simulink library "csu_itu_inertial_time_update_lib"  (R2014b)
settings: Solver=ode45  SolverMode=SingleTasking  StartTime=0.0  StopTime=10.0  RelTol=1e-3
values from neighbouring files (symbols this model uses):
  tup_process_noise_high = diag([1.1 1.1 10.1 , 0.000505   0.000505   0.000505 ,  0.00001 0.00001 0.00001 , 0.001 0.001 0.001 , 0.001 0.001 0.001 ])    [csc_tup_time_update_init.m]
undefined symbols (not defined in the file or in its folder): est_time_step, kfl_gibbs_index, tup_state_update_init
libraries: util_quat_lib x2, util_info_lib x1, util_common_lib x1
settings Model: ExtModeAutoUpdateStatusClock=off  Creator=escrane  LastModifiedBy=mstewart

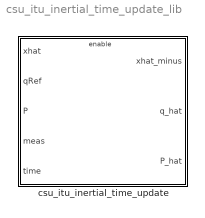
== system csu_itu_inertial_time_update_lib ==
  csu_itu_inertial_time_update : Subsystem

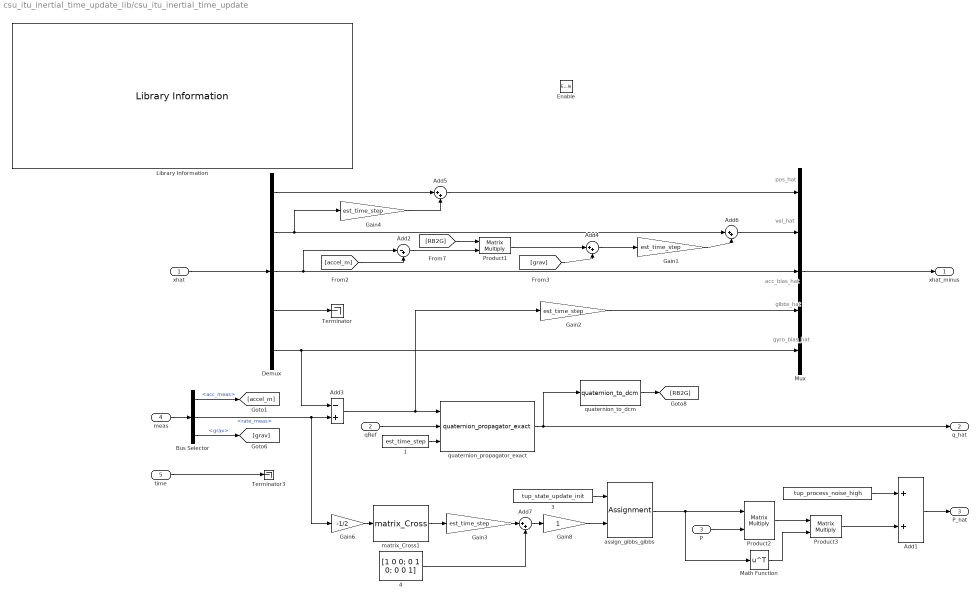
== system csu_itu_inertial_time_update_lib/csu_itu_inertial_time_update ==
  note: gyro_bias_hat
  note: gibbs_hat
  note: acc_bias_hat
  note: vel_hat
  note: pos_hat
  xhat : Inport
  qRef : Inport  Port=2
  P : Inport  Port=3
  meas : Inport  Port=4
  time : Inport  Port=5
  Enable : EnablePort  StatesWhenEnabling=reset
  "      " : Constant  Value=tup_process_noise_high
  "      1" : Constant  Value=est_time_step
  "      3" : Constant  Value=tup_state_update_init
  "      4" : Constant  Value=[1 0 0; 0 1 0; 0 0 1]
  Add1 : Sum
  Add2 : Sum  Inputs=|-+
  Add3 : Sum  Inputs=-+
  Add{4..7} (4 alike) : Sum  Inputs=|++
  Bus Selector : BusSelector  OutputSignals=acc_meas,rate_meas,grav
  Demux : Demux  Outputs=[3 3 3 3 3]
  Gain{1..4} (4 alike) : Gain  Gain=est_time_step
  Gain6 : Gain  Gain=-1/2
  Gain8 : Gain
  Library Information : util_info_lib/Library Information  owner='escrane'
  Math Function : Math  Operator=transpose  SaturateOnIntegerOverflow=on
  Mux : Mux  Inputs=5
  Product1 : Product  Multiplication=Matrix(*)  RndMeth=Zero  InputSameDT=on
  Product2 : Product  Multiplication=Matrix(*)  RndMeth=Zero  InputSameDT=on
  Product3 : Product  Multiplication=Matrix(*)  RndMeth=Zero  InputSameDT=on
  Terminator : Terminator
  Terminator3 : Terminator
  assign_gibbs_gibbs : Assignment  NumberOfDimensions=2  IndexOptions=Index vector (dialog),Index vector (dialog)  Indices=kfl_gibbs_index,kfl_gibbs_index  OutputSizes=1,1
  matrix_Cross1 : util_common_lib/matrix_Cross  SystemSampleTime=-1
  quaternion_propagator_exact : util_quat_lib/quaternion_propagator_exact  SystemSampleTime=-1
  quaternion_to_dcm : util_quat_lib/quaternion_to_dcm  SystemSampleTime=-1
  xhat_minus : Outport
  q_hat : Outport  Port=2
  P_hat : Outport  Port=3
  wires:
  Gain8/1 -> assign_gibbs_gibbs/2
  Gain3/1 -> Add7/1
  Gain6/1 -> matrix_Cross1/1
  Add7/1 -> Gain8/1
  "      4"/1 -> Add7/2
  matrix_Cross1/1 -> Gain3/1
  Add3/1 -> quaternion_propagator_exact/1, Gain2/1
  "      3"/1 -> assign_gibbs_gibbs/1
  Add1/1 -> P_hat/1
  Product3/1 -> Add1/2
  "      "/1 -> Add1/1
  Math Function/1 -> Product3/2
  Product2/1 -> Product3/1
  P/1 -> Product2/2
  assign_gibbs_gibbs/1 -> Product2/1, Math Function/1
  Bus Selector/2 -> Add3/2, Gain6/1  "<rate_meas>"
  meas/1 -> Bus Selector/1
  Bus Selector/1 -> [accel_m]  "<acc_meas>"
  Demux/5 -> Mux/5, Add3/1
  Add4/1 -> Gain1/1
  [grav] -> Add4/2
  Product1/1 -> Add4/1
  Gain2/1 -> Mux/4
  [RB2G] -> Product1/1
  quaternion_to_dcm/1 -> [RB2G]
  Add6/1 -> Mux/2
  Add5/1 -> Mux/1
  Gain1/1 -> Add6/2
  Gain4/1 -> Add5/2
  "      1"/1 -> quaternion_propagator_exact/3
  qRef/1 -> quaternion_propagator_exact/2
  quaternion_propagator_exact/1 -> q_hat/1, quaternion_to_dcm/1
  Add2/1 -> Product1/2
  [accel_m] -> Add2/2
  Demux/3 -> Add2/1, Mux/3
  Demux/2 -> Add6/1, Gain4/1
  Demux/1 -> Add5/1
  Demux/4 -> Terminator/1
  Mux/1 -> xhat_minus/1
  xhat/1 -> Demux/1
  Bus Selector/3 -> [grav]  "<grav>"
  time/1 -> Terminator3/1
